simulink model "Problem2"  (R2020b)
settings: Solver=VariableStepAuto  StartTime=0.0  StopTime=100  RelTol=1e-3
PreLoadFcn:
  | clear all;
  | close all;
  | clc;
  | th=linspace(0,3*pi);
  | r=0.1*sin(th);
  | r(th>pi)=0;
  | m2=50;
  | k1=5700;
  | k2=135000;
  | b=290;
  | F=1;
  | m1=100;
model workspace (MAT data in the model file):
  F = Simulink.Parameter
  F.Value = 1
  F.DataType = 'auto'
  F.Dimensions = [1 1]
  Param = Simulink.Parameter
  Param.DataType = 'auto'
  Param.Dimensions = [0 0]
  b = Simulink.Parameter
  b.Value = 290
  b.DataType = 'auto'
  b.Dimensions = [1 1]
  k1 = Simulink.Parameter
  k1.Value = 5700
  k1.DataType = 'auto'
  k1.Dimensions = [1 1]
  k2 = Simulink.Parameter
  k2.Value = 135000
  k2.DataType = 'auto'
  k2.Dimensions = [1 1]
  m1 = Simulink.Parameter
  m1.Value = 100
  m1.DataType = 'auto'
  m1.Dimensions = [1 1]
  m2 = Simulink.Parameter
  m2.Value = 50
  m2.DataType = 'auto'
  m2.Dimensions = [1 1]
  r = Simulink.Parameter
  r.Value = [0 0.00950560433042 0.018925124436 0.0281732556841 0.037166245566 0.0458226521727 0.0540640817456 0.0618158986221 0.0690079011482 0.0755749574354 0.081457595205 0.0866025403784 0.0909631995355 0.0945000818715 0.0971811568324 0.0989821441881 0.0998867339183 0.0998867339183 0.0989821441881 0.0971811568324 0.0945000818715 0.0909631995355 0.0866025403784 0.081457595205 0.0755749574354 0.0690079011482 0.0618158986221 0.0540640817456 0.0458226521727 0.037166245566 0.0281732556841 0.018925124436 0.00950560433042 0 0 0 0 0 0 0 0 0 0 0 0 0 0 0 0 0 0 0 0 0 0 0 0 0 0 0 0 0 0 0 0 0 0 0 0 0 0 0 0 0 0 0 0 0 0 0 0 0 0 0 0 0 0 0 0 0 0 0 0 0 0 0 0 0 0 0]
  r.DataType = 'auto'
  r.Dimensions = [1 100]
  th = Simulink.Parameter
  th.Value = [0 0.0951997773815 0.190399554763 0.285599332145 0.380799109526 0.475998886908 0.571198664289 0.666398441671 0.761598219052 0.856797996434 0.951997773815 1.0471975512 1.14239732858 1.23759710596 1.33279688334 1.42799666072 1.5231964381 1.61839621549 1.71359599287 1.80879577025 1.90399554763 1.99919532501 2.09439510239 2.18959487977 2.28479465716 2.37999443454 2.47519421192 2.5703939893 2.66559376668 2.76079354406 2.85599332145 2.95119309883 3.04639287621 3.14159265359 3.23679243097 3.33199220835 3.42719198573 3.52239176312 3.6175915405 3.71279131788 3.80799109526 3.90319087264 3.99839065002 4.0935904274 4.18879020479 4.28398998217 4.37918975955 4.47438953693 4.56958931431 4.66478909169 4.75998886908 4.85518864646 4.95038842384 5.04558820122 5.1407879786 5.23598775598 5.33118753336 5.42638731075 5.52158708813 5.61678686551 5.71198664289 5.80718642027 5.90238619765 5.99758597504 6.09278575242 6.1879855298 6.28318530718 6.37838508456 6.47358486194 6.56878463932 6.66398441671 6.75918419409 6.85438397147 6.94958374885 7.04478352623 7.13998330361 7.23518308099 7.33038285838 7.42558263576 7.52078241314 7.61598219052 7.7111819679 7.80638174528 7.90158152267 7.99678130005 8.09198107743 8.18718085481 8.28238063219 8.37758040957 8.47278018695 8.56797996434 8.66317974172 8.7583795191 8.85357929648 8.94877907386 9.04397885124 9.13917862862 9.23437840601 9.32957818339 9.42477796077]
  th.DataType = 'auto'
  th.Dimensions = [1 100]
settings Model: OrderedModelArguments=off  Creator=amolg  LastModifiedBy=amolg

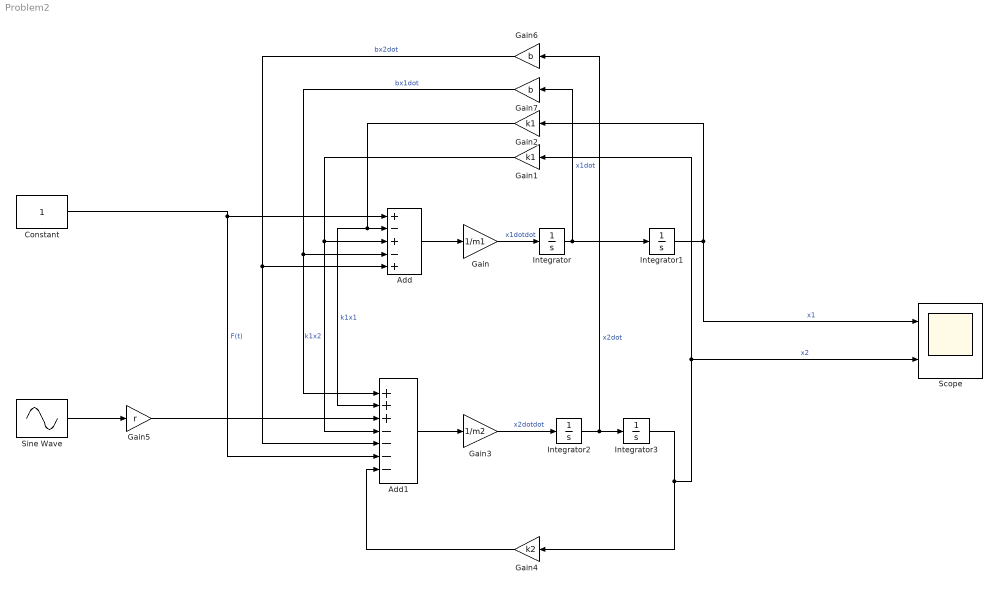
== system Problem2 ==
  Add : Sum  Inputs=+-+-+
  Add1 : Sum  Inputs=+++----
  Constant : Constant
  Gain : Gain  Gain=1/m1
  Gain1 : Gain  Gain=k1
  Gain2 : Gain  Gain=k1
  Gain3 : Gain  Gain=1/m2
  Gain4 : Gain  Gain=k2
  Gain5 : Gain  Gain=r
  Gain6 : Gain  Gain=b
  Gain7 : Gain  Gain=b
  Integrator{,1..3} (4 alike) : Integrator
  Scope : Scope  NumInputPorts=2
  Sine Wave : Sin  SampleTime=0
  wires:
  Gain2/1 -> Add1/2, Add/2  "k1x1"
  Gain1/1 -> Add1/4, Add/3  "k1x2"
  Gain4/1 -> Add1/7
  Gain7/1 -> Add/4, Add1/1  "bx1dot"
  Sine Wave/1 -> Gain5/1
  Constant/1 -> Add1/6, Add/1  "F(t)"
  Integrator3/1 -> Gain4/1, Gain1/1, Scope/2  "x2"
  Gain3/1 -> Integrator2/1  "x2dotdot"
  Gain/1 -> Integrator/1  "x1dotdot"
  Gain6/1 -> Add1/5, Add/5  "bx2dot"
  Integrator1/1 -> Scope/1, Gain2/1  "x1"
  Add1/1 -> Gain3/1
  Gain5/1 -> Add1/3
  Integrator/1 -> Gain7/1, Integrator1/1  "x1dot"
  Integrator2/1 -> Gain6/1, Integrator3/1  "x2dot"
  Add/1 -> Gain/1
